simulink model "modulator"  (R2024b)
settings: Solver=ode1be  StartTime=0.0  StopTime=simlength  FixedStep=tc  MaxStep=tc
undefined symbols (not defined in the file or in its folder): ts_afe
settings Model: Creator=dbagn  LastModifiedBy=dbagn
settings SolverCC: NumberNewtonIterations=3  ZeroCrossControl=DisableAll  AlgebraicLoopSolver=TrustRegion  SolverResetMethod=Robust
settings DataIOCC: ReturnWorkspaceOutputs=off
settings OptimizationCC: ReuseModelBlockBuffer=off
settings DebuggingCC: UnconnectedInputMsg=warning  UnconnectedOutputMsg=warning  UnconnectedLineMsg=warning
settings ModelReferenceCC: EnableRefExpFcnMdlSchedulingChecks=on
settings SFSimCC: CustomCodeUndefinedFunction=ThrowError
settings SFSimCC: SimCustomHeaderCode=|
  | #include "math_f.h"
  | #include "mavgflt.h"
  | #include "mavgflt_simulink.h"
  | #include "bemf_obsv.h"
  | #include "bemf_obsv_simulink.h"
  | #include "bemf_obsv_load_est.h"
  | #include "bemf_obsv_load_est_simulink.h"
  | #include "bemf_obsv_redu.h"
  | #include "bemf_obsv_redu_simulink.h"
  | #include "bemf_obsv_load_est_redu.h"
  | #include "bemf_obsv_load_est_redu_simulink.h"
  | #include "dqvector_pi.h"
  | #include "dqvector_pi_simulink.h"
  | #include "sv_pwm_simulink.h"
  | #include "sv_pwm.h"
settings SFSimCC: SimUserSources=|
  | "mavgflt_simulink.c"
  | "mavgflt.c"
  | "bemf_obsv_simulink.c"
  | "bemf_obsv.c"
  | "bemf_obsv_load_est_simulink.c"
  | "bemf_obsv_load_est.c"
  | "bemf_obsv_redu_simulink.c"
  | "bemf_obsv_redu.c"
  | "bemf_obsv_load_est_redu_simulink.c"
  | "bemf_obsv_load_est_redu.c"
  | "dqvector_pi.c"
  | "dqvector_pi_simulink.c"
  | "sv_pwm_simulink.c"
  | "sv_pwm.c"
settings SFSimCC: SimUserIncludeDirs=|
  | include
  | src
settings RTWCC: GPUComputeCapability=3.5  DLArmComputeVersion=19.05

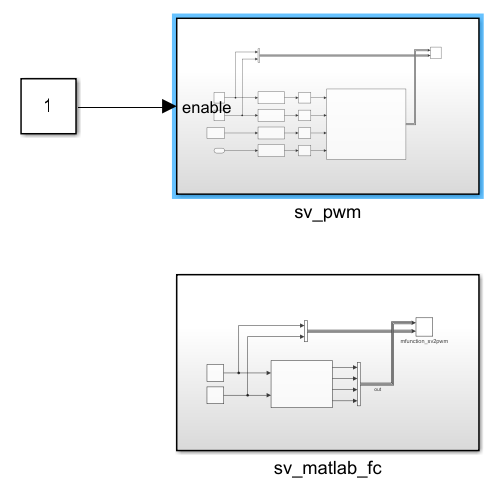
[thumbnail: Simulink's stored preview of the top-level diagram]
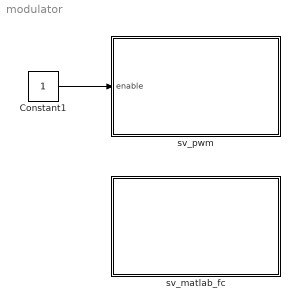
== system modulator ==
  Constant1 : Constant
  sv_matlab_fc : Subsystem
  sv_pwm : Subsystem
  wires:
  Constant1/1 -> sv_pwm/1(enable)

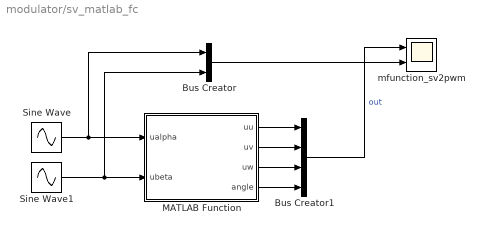
== system modulator/sv_matlab_fc ==
  Bus Creator : BusCreator  Inputs=2
  Bus Creator1 : BusCreator  Inputs=4
  MATLAB Function : MATLAB Function  TreatAsAtomicUnit=on  SystemSampleTime=ts_afe
  Sine Wave : Sin  Amplitude=sqrt(3)/2  Frequency=2*pi*50  SampleTime=0
  Sine Wave1 : Sin  Amplitude=sqrt(3)/2  Frequency=2*pi*50  Phase=-pi/2  SampleTime=0
  mfunction_sv2pwm : Scope  NumInputPorts=2
  wires:
  Bus Creator/1 -> mfunction_sv2pwm/2
  Bus Creator1/1 -> mfunction_sv2pwm/1  "out"
  Sine Wave1/1 -> MATLAB Function/2(ubeta), Bus Creator/2
  Sine Wave/1 -> MATLAB Function/1(ualpha), Bus Creator/1
  MATLAB Function/3(uw) -> Bus Creator1/3
  MATLAB Function/2(uv) -> Bus Creator1/2
  MATLAB Function/1(uu) -> Bus Creator1/1
  MATLAB Function/4(angle) -> Bus Creator1/4

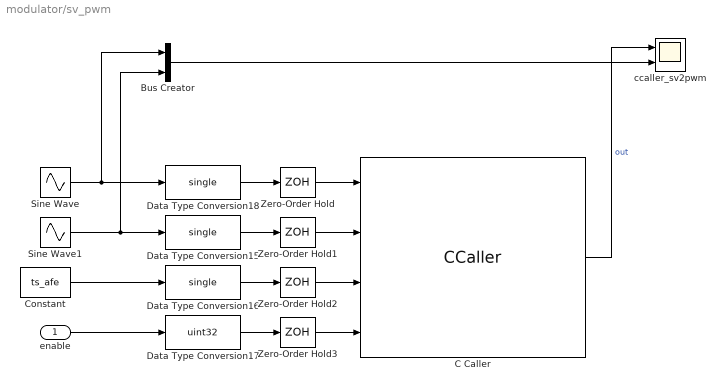
== system modulator/sv_pwm ==
  enable : Inport
  Bus Creator : BusCreator  Inputs=2
  C Caller : CCaller  FunctionName=sv_pwm_process_simulink  PortSpecificationStruct="%)30     .    V @   8    (     @         %    \"     4    !     0         %  0 \"0    $    _    07)G3F%M90  4&]R=$YA;64 4V-O<&4     26YD97@     5'EP90      4VEZ90      27-';&]B86P   X    P    !@    @    $          4    (     0    ,    !         !   P!O=70 #@   #     &    \"     0         !0    @    !     P    $         $  # &]U=  .    .     8    (    !          %    \"     $    &     0         0   ...(+2669 chars)"  SampleTime=ts_afe
  Constant : Constant  Value=ts_afe
  Data Type Conversion15 : DataTypeConversion  OutDataTypeStr=single  SaturateOnIntegerOverflow=off  RndMeth=Floor
  Data Type Conversion16 : DataTypeConversion  OutDataTypeStr=single  SaturateOnIntegerOverflow=off  RndMeth=Floor
  Data Type Conversion17 : DataTypeConversion  OutDataTypeStr=uint32  SaturateOnIntegerOverflow=off  RndMeth=Floor
  Data Type Conversion18 : DataTypeConversion  OutDataTypeStr=single  SaturateOnIntegerOverflow=off  RndMeth=Floor
  Sine Wave : Sin  Amplitude=sqrt(3)/2  Frequency=2*pi*50  SampleTime=0
  Sine Wave1 : Sin  Amplitude=sqrt(3)/2  Frequency=2*pi*50  Phase=pi/2  SampleTime=0
  Zero-Order Hold{,1..3} (4 alike) : ZeroOrderHold  SampleTime=ts_afe
  ccaller_sv2pwm : Scope  NumInputPorts=2
  wires:
  Zero-Order Hold2/1 -> C Caller/3
  Constant/1 -> Data Type Conversion16/1
  Data Type Conversion18/1 -> Zero-Order Hold/1
  enable/1 -> Data Type Conversion17/1
  Data Type Conversion16/1 -> Zero-Order Hold2/1
  Data Type Conversion17/1 -> Zero-Order Hold3/1
  Zero-Order Hold3/1 -> C Caller/4
  Data Type Conversion15/1 -> Zero-Order Hold1/1
  Zero-Order Hold/1 -> C Caller/1
  Zero-Order Hold1/1 -> C Caller/2
  C Caller/1 -> ccaller_sv2pwm/1  "out"
  Sine Wave/1 -> Bus Creator/1, Data Type Conversion18/1
  Sine Wave1/1 -> Bus Creator/2, Data Type Conversion15/1
  Bus Creator/1 -> ccaller_sv2pwm/2

== matlab function modulator/sv_matlab_fc/MATLAB Function ==
  data: ualpha input; uu output; ubeta input; uv output; uw output; angle output
function [uu, uv, uw, angle] = sv(ualpha, ubeta)

persistent ua ub uc t0 t1 t2;
if isempty(ua)
    ua = 0;
    ub = 0;
    uc = 0;
    t0 = 0;
    t1 = 0;
    t2 = 0;
end
    angle = atan2(ubeta,ualpha);
    
    if (angle >= 0 && angle <= pi/3)
        % sector1 (counterclockwise)
        t2 = ubeta*2/sqrt(3); %v2
        t1 = ualpha - ubeta/sqrt(3); %v1
        t0 = 1 - t2 - t1;
        ua = t0/2;
        ub = t1 + ua;
        uc = t2 + ub;
    end
    if (angle >= pi/3 && angle <= 2*pi/3)
        % sector2 (clockwise)
        t1 = -ualpha + ubeta/sqrt(3); %v3
        t2 = ualpha + ubeta/sqrt(3); %v2
        t0 = 1 - t2 - t1;
        ub = t0/2;
        ua = t1 + ub;
        uc = t2 + ua;
    end
    if (angle >= 2*pi/3 && angle <= pi)
        % sector3 (counterclockwise)
        t2 = -ubeta/sqrt(3) - ualpha; %v4
        t1 = ubeta*2/sqrt(3); %v3
        t0 = 1 - t2 - t1;
        ub = t0/2;
        uc = t1 + ub;
        ua = t2 + uc;
    end
    if (angle >= -pi && angle <= -2*pi/3)
        % sector4 (clockwise)
        t1 = -2/sqrt(3)*ubeta; %v5
        t2 = ubeta/sqrt(3) - ualpha; %v4
        t0 = 1 - t2 - t1;
        uc = t0/2;
        ub = t1 + uc;
        ua = t2 + ub;
    end

    if (angle >= -2*pi/3 && angle <= -pi/3)
        % sector5 (counterclockwise)
        t2 = ualpha - 1/sqrt(3)*ubeta; %v6
        t1 = -ualpha - 1/sqrt(3)*ubeta; %v5
        t0 = 1 - t2 - t1;
        uc = t0/2;
        ua = t1 + uc;
        ub = t2 + ua;
    end
    if (angle >= -pi/3 && angle <= 0)
        % sector6 (clockwise)
        t1 = ualpha + ubeta/sqrt(3); %v1
        t2 = -ubeta*2/sqrt(3); %v6
        t0 = 1 - t2 - t1;
        ua = t0/2;
        uc = t1 + ua;
        ub = t2 + uc;
    end

uu = ua;
uv = ub;
uw = uc;
